simulink model "BEncoderError"  (R2024b)
settings: configuration reference "STM32H7_Config" (kept outside this file)
libraries: simulink x8
settings Model: DataDictionary=Master_Dictionary.sldd  EnableAccessToBaseWorkspace=off  Creator=torni  LastModifiedBy=William
settings ConfigSetRef: SourceName=STM32H7_Config

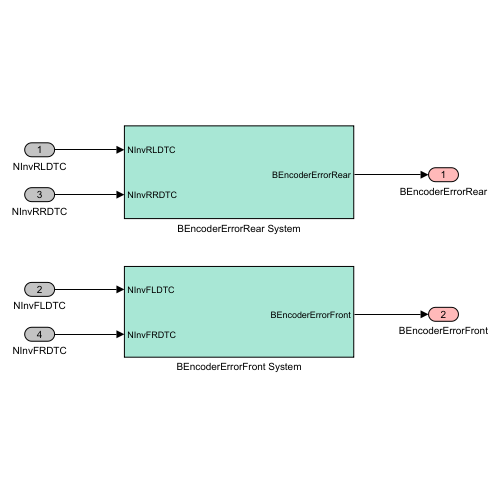
[thumbnail: Simulink's stored preview of the top-level diagram]
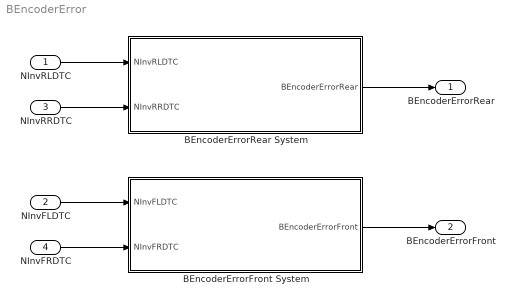
== system BEncoderError ==
  NInvRLDTC : Inport  OutDataTypeStr=double
  NInvFLDTC : Inport  Port=2  OutDataTypeStr=double
  NInvRRDTC : Inport  Port=3  OutDataTypeStr=double
  NInvFRDTC : Inport  Port=4  OutDataTypeStr=double
  BEncoderErrorFront System : Subsystem
  BEncoderErrorRear System : Subsystem
  BEncoderErrorRear : Outport  OutDataTypeStr=boolean  VectorParamsAs1DForOutWhenUnconnected=off
  BEncoderErrorFront : Outport  Port=2  OutDataTypeStr=boolean  VectorParamsAs1DForOutWhenUnconnected=off
  wires:
  BEncoderErrorFront System/1(BEncoderErrorFront) -> BEncoderErrorFront/1
  NInvRRDTC/1 -> BEncoderErrorRear System/2(NInvRRDTC)
  NInvFLDTC/1 -> BEncoderErrorFront System/1(NInvFLDTC)
  BEncoderErrorRear System/1(BEncoderErrorRear) -> BEncoderErrorRear/1
  NInvFRDTC/1 -> BEncoderErrorFront System/2(NInvFRDTC)
  NInvRLDTC/1 -> BEncoderErrorRear System/1(NInvRLDTC)

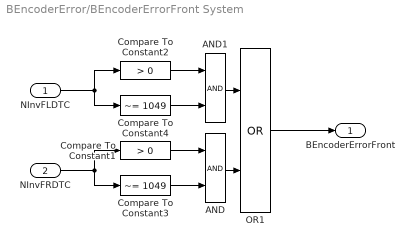
== system BEncoderError/BEncoderErrorFront System ==
  NInvFLDTC : Inport  OutDataTypeStr=double
  NInvFRDTC : Inport  Port=2  OutDataTypeStr=double
  AND : Logic  AllPortsSameDT=off  OutDataTypeStr=boolean
  AND1 : Logic  AllPortsSameDT=off  OutDataTypeStr=boolean
  Compare To Constant1 : simulink/Logic and Bit Operations/Compare To Constant  relop=>  const=0  OutDataTypeStr=boolean
  Compare To Constant2 : simulink/Logic and Bit Operations/Compare To Constant  relop=>  const=0  OutDataTypeStr=boolean
  Compare To Constant3 : simulink/Logic and Bit Operations/Compare To Constant  relop=~=  const=1049  OutDataTypeStr=boolean
  Compare To Constant4 : simulink/Logic and Bit Operations/Compare To Constant  relop=~=  const=1049  OutDataTypeStr=boolean
  OR1 : Logic  Operator=OR  AllPortsSameDT=off  OutDataTypeStr=boolean
  BEncoderErrorFront : Outport  OutDataTypeStr=boolean  VectorParamsAs1DForOutWhenUnconnected=off
  wires:
  OR1/1 -> BEncoderErrorFront/1
  Compare To Constant2/1 -> AND1/1
  Compare To Constant1/1 -> AND/1
  NInvFLDTC/1 -> Compare To Constant2/1, Compare To Constant4/1
  Compare To Constant3/1 -> AND/2
  Compare To Constant4/1 -> AND1/2
  NInvFRDTC/1 -> Compare To Constant3/1, Compare To Constant1/1
  AND1/1 -> OR1/1
  AND/1 -> OR1/2

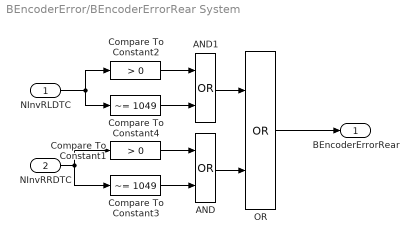
== system BEncoderError/BEncoderErrorRear System ==
  NInvRLDTC : Inport  OutDataTypeStr=double
  NInvRRDTC : Inport  Port=2  OutDataTypeStr=double
  AND : Logic  Operator=OR  AllPortsSameDT=off  OutDataTypeStr=boolean
  AND1 : Logic  Operator=OR  AllPortsSameDT=off  OutDataTypeStr=boolean
  Compare To Constant1 : simulink/Logic and Bit Operations/Compare To Constant  relop=>  const=0  OutDataTypeStr=boolean
  Compare To Constant2 : simulink/Logic and Bit Operations/Compare To Constant  relop=>  const=0  OutDataTypeStr=boolean
  Compare To Constant3 : simulink/Logic and Bit Operations/Compare To Constant  relop=~=  const=1049  OutDataTypeStr=boolean
  Compare To Constant4 : simulink/Logic and Bit Operations/Compare To Constant  relop=~=  const=1049  OutDataTypeStr=boolean
  OR : Logic  Operator=OR  AllPortsSameDT=off  OutDataTypeStr=boolean
  BEncoderErrorRear : Outport  OutDataTypeStr=boolean  VectorParamsAs1DForOutWhenUnconnected=off
  wires:
  OR/1 -> BEncoderErrorRear/1
  AND1/1 -> OR/1
  Compare To Constant3/1 -> AND/2
  AND/1 -> OR/2
  Compare To Constant1/1 -> AND/1
  NInvRRDTC/1 -> Compare To Constant3/1, Compare To Constant1/1
  Compare To Constant2/1 -> AND1/1
  Compare To Constant4/1 -> AND1/2
  NInvRLDTC/1 -> Compare To Constant4/1, Compare To Constant2/1
